simulink model "debugging_task"  (Simulink 3.0)
libraries: genlib x5, logiclib x5, speclib x1

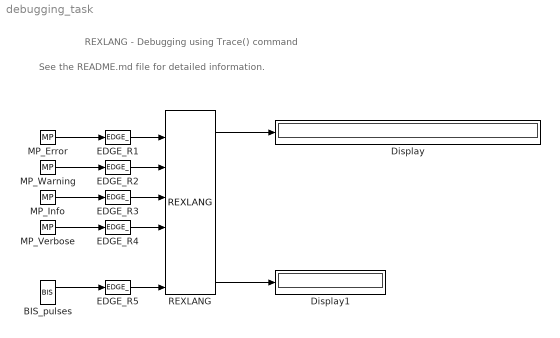
== system debugging_task ==
  note: See the README.md file for detailed information.
  note: REXLANG - Debugging using Trace() command
  BIS_pulses : genlib/BIS  Y0=off  t1=1  t2=2  t3=0  t4=4  t5=5  t6=6  t7=7  t8=8  RPT=on
  Display : Display
      settings: Format=Best fit
  Display1 : Display
      settings: Format=Best fit  Suffix=pulses
  EDGE_R{1..5} (5 alike) : logiclib/EDGE_  iedge=1: Rising edge
  MP_Error : genlib/MP  BSTATE=off  pwidth=0.2  RPTF=off
  MP_Info : genlib/MP  BSTATE=off  pwidth=0.2  RPTF=off
  MP_Verbose : genlib/MP  BSTATE=off  pwidth=0.2  RPTF=off
  MP_Warning : genlib/MP  BSTATE=off  pwidth=0.2  RPTF=off
  REXLANG : speclib/REXLANG  strs=0  SystemSampleTime=-1  tab_matlab=BASIC  srcname=debugging_rexlang.c  srctype=1: C-like  stack=0  debug=1: No check  p0=2.6  p1=8.9  p2=0  p3=0  p4=0  p5=0  p6=0  p7=0  p8=0  p9=0  p10=0  p11=0  p12=0  p13=0  p14=0  p15=0
  wires:
  BIS_pulses/1 -> EDGE_R5/1
  EDGE_R1/1 -> REXLANG/3
  EDGE_R2/1 -> REXLANG/6
  EDGE_R3/1 -> REXLANG/9
  EDGE_R4/1 -> REXLANG/12
  EDGE_R5/1 -> REXLANG/18
  MP_Error/1 -> EDGE_R1/1
  MP_Info/1 -> EDGE_R3/1
  MP_Verbose/1 -> EDGE_R4/1
  MP_Warning/1 -> EDGE_R2/1
  REXLANG/2 -> Display/1
  REXLANG/17 -> Display1/1
